simulink model "sun_point_unit_test"  (R2016b)
settings: Solver=VariableStepAuto  StartTime=0.0  StopTime=1000  MaxStep=0.01  RelTol=1e-4  EnableMultiTasking=on
undefined symbols (not defined in the file): fsw_params, sun_point_lib
libraries: aerolibutil x6, dspmathops x3, simulink x2
settings Model: Creator=Krish  LastModifiedBy=Taylor
settings DataIOCC: LimitDataPoints=on  SaveOutput=off  SaveTime=off
settings OptimizationCC: ExpressionDepthLimit=2147483647  LifeSpan=1
settings DebuggingCC: UnderspecifiedInitializationDetection=Classic  MergeDetectMultiDrivingBlocksExec=none  FcnCallInpInsideContextMsg=warning  AllowSymbolicDim=off  StateNameClashWarn=warning  SFUnexpectedBacktrackingDiag=warning  SFNoUnconditionalDefaultTransitionDiag=warning  SFExecutionAtInitializationDiag=none
settings GRTTargetCC: TargetLangStandard=C89/C90 (ANSI)  GeneratePreprocessorConditionals=Disable all  CombineOutputUpdateFcns=off  GRTInterface=on

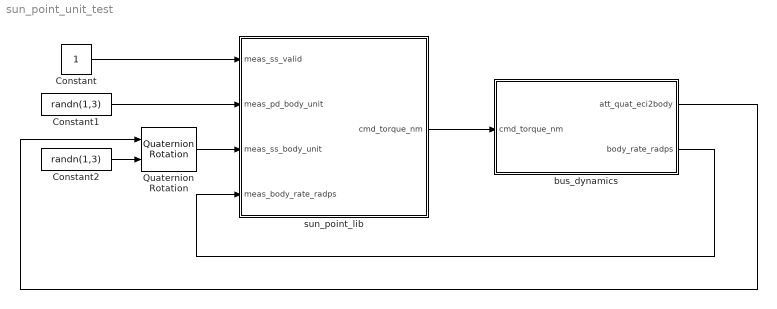
== system sun_point_unit_test ==
  Constant : Constant
  Constant1 : Constant  Value=randn(1,3)
  Constant2 : Constant  Value=randn(1,3)
  Quaternion Rotation : aerolibutil/Quaternion Rotation
  bus_dynamics : Subsystem
  sun_point_lib : Subsystem  AncestorBlock=sun_point_lib/sun_point_lib  TreatAsAtomicUnit=on
      settings: MinAlgLoopOccurrences=on  RTWFcnNameOpts=Use subsystem name  RTWFileNameOpts=Use subsystem name
  wires:
  sun_point_lib/1(cmd_torque_nm) -> bus_dynamics/1(cmd_torque_nm)
  Constant/1 -> sun_point_lib/1(meas_ss_valid)
  Constant1/1 -> sun_point_lib/2(meas_pd_body_unit)
  Quaternion Rotation/1 -> sun_point_lib/3(meas_ss_body_unit)
  Constant2/1 -> Quaternion Rotation/2
  bus_dynamics/1(att_quat_eci2body) -> Quaternion Rotation/1
  bus_dynamics/2(body_rate_radps) -> sun_point_lib/4(meas_body_rate_radps)

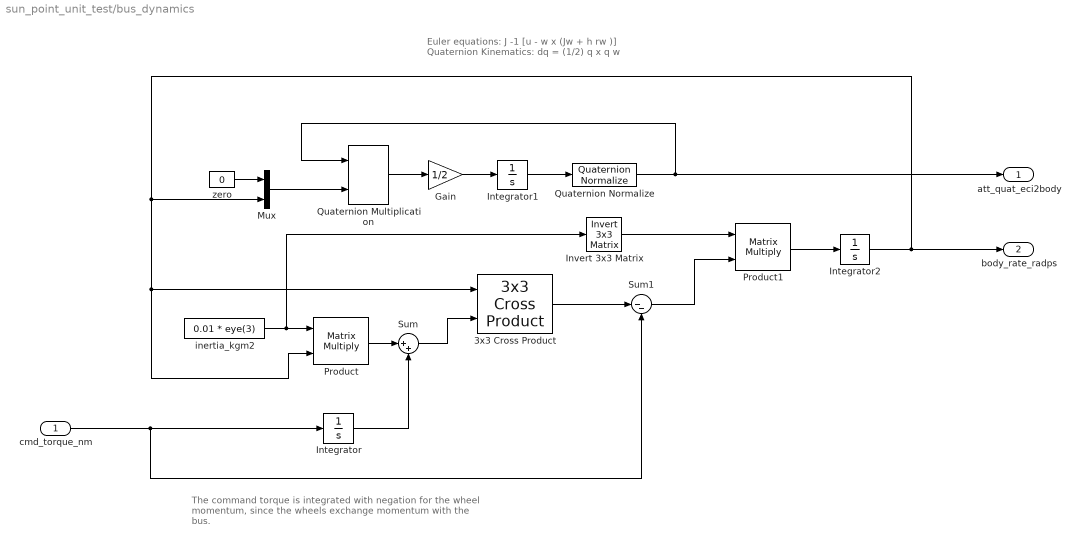
== system sun_point_unit_test/bus_dynamics ==
  note: Euler equations: J -1 [u - w x (Jw + h rw )]
      | Quaternion Kinematics: dq = (1/2) q x q w
  note: The command torque is integrated with negation for the wheel
      | momentum, since the wheels exchange momentum with the bus.
  cmd_torque_nm : Inport
  3x3 Cross Product : aerolibutil/3x3 Cross Product
  Gain : Gain  Gain=1/2
  Integrator : Integrator  InitialCondition=[0 0 0]
      settings: AttributesFormatString=IC: %<InitialCondition>
  Integrator1 : Integrator  InitialCondition=[1 0 0 0]
      settings: AttributesFormatString=IC: %<InitialCondition>
  Integrator2 : Integrator  InitialCondition=[0 0 0]
      settings: AttributesFormatString=IC: %<InitialCondition>
  Invert 3x3 Matrix : aerolibutil/Invert  3x3 Matrix
  Mux : Mux  Inputs=[1 3]
  Product : Product  Multiplication=Matrix(*)
  Product1 : Product  Multiplication=Matrix(*)
  Quaternion Multiplication : aerolibutil/Quaternion Multiplication
  Quaternion Normalize : aerolibutil/Quaternion Normalize
  Sum : Sum  Inputs=|++
  Sum1 : Sum  Inputs=|--
  inertia_kgm2 : Constant  Value=0.01 * eye(3)
  zero : Constant  Value=0
  att_quat_eci2body : Outport
  body_rate_radps : Outport  Port=2
  wires:
  Quaternion Normalize/1 -> att_quat_eci2body/1, Quaternion Multiplication/1
  Integrator2/1 -> body_rate_radps/1, 3x3 Cross Product/1, Product/2, Mux/2
  Product/1 -> Sum/1
  Sum/1 -> 3x3 Cross Product/2
  Integrator/1 -> Sum/2
  3x3 Cross Product/1 -> Sum1/1
  Integrator1/1 -> Quaternion Normalize/1
  zero/1 -> Mux/1
  Mux/1 -> Quaternion Multiplication/2
  Quaternion Multiplication/1 -> Gain/1
  Gain/1 -> Integrator1/1
  inertia_kgm2/1 -> Invert 3x3 Matrix/1, Product/1
  Invert 3x3 Matrix/1 -> Product1/1
  Sum1/1 -> Product1/2
  Product1/1 -> Integrator2/1
  cmd_torque_nm/1 -> Integrator/1, Sum1/2

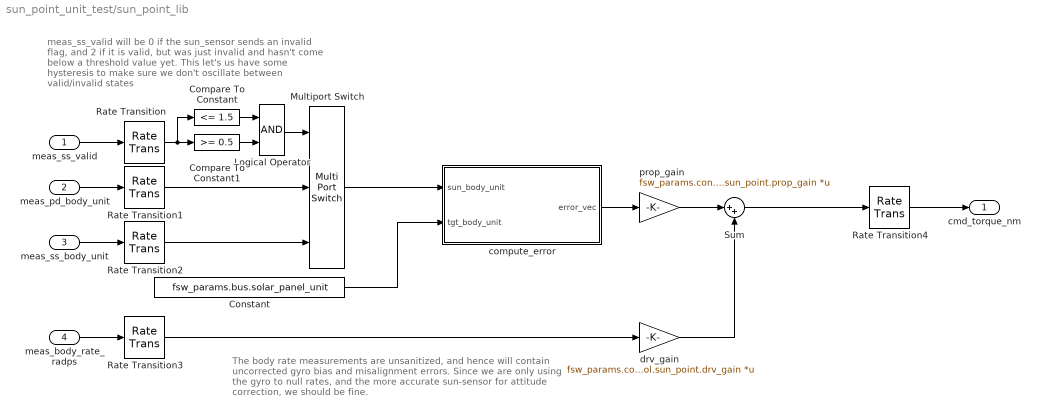
== system sun_point_unit_test/sun_point_lib ==
  note: The body rate measurements are unsanitized, and hence will contain
      | uncorrected gyro bias and misalignment errors. Since we are only using
      | the gyro to null rates, and the more accurate sun-sensor for attitude
      | correction, we should be fine.
  note: meas_ss_valid will be 0 if the sun_sensor sends an
      | invalid flag, and 2 if it is valid, but was just
      | invalid and hasn't come below a threshold value yet.
      | This let's us have some hysteresis to make sure we don't
      | oscillate between valid/invalid states
  meas_ss_valid : Inport
  meas_pd_body_unit : Inport  Port=2
  meas_ss_body_unit : Inport  Port=3
  meas_body_rate_radps : Inport  Port=4
  Compare To Constant : simulink/Logic and Bit Operations/Compare To Constant  relop=<=  const=1.5  OutDataTypeStr=boolean
  Compare To Constant1 : simulink/Logic and Bit Operations/Compare To Constant  relop=>=  const=0.5  OutDataTypeStr=boolean
  Constant : Constant  Value=fsw_params.bus.solar_panel_unit
  Logical Operator : Logic  AllPortsSameDT=off  OutDataTypeStr=boolean
  Multiport Switch : MultiPortSwitch  DataPortOrder=Zero-based contiguous  Inputs=2
  Rate Transition : RateTransition  X0=fsw_params.control.sun_point.ic.meas_ss_valid  OutPortSampleTime=fsw_params.control.sun_point.sample_time_s
  Rate Transition1 : RateTransition  X0=fsw_params.control.sun_point.ic.meas_pd_body_unit  OutPortSampleTime=fsw_params.control.sun_point.sample_time_s
  Rate Transition2 : RateTransition  X0=fsw_params.control.sun_point.ic.meas_ss_body_unit  OutPortSampleTime=fsw_params.control.sun_point.sample_time_s
  Rate Transition3 : RateTransition  X0=fsw_params.control.sun_point.ic.meas_body_rate_radps  OutPortSampleTime=fsw_params.control.sun_point.sample_time_s
  Rate Transition4 : RateTransition  X0=fsw_params.control.sun_point.ic.cmd_torque_nm  OutPortSampleTimeOpt=Inherit
  Sum : Sum  Inputs=|++
  compute_error : Subsystem
  drv_gain : Gain  Gain=fsw_params.control.sun_point.drv_gain  Multiplication=Matrix(K*u)
  prop_gain : Gain  Gain=fsw_params.control.sun_point.prop_gain  Multiplication=Matrix(K*u)
  cmd_torque_nm : Outport
  wires:
  Logical Operator/1 -> Multiport Switch/1
  Compare To Constant1/1 -> Logical Operator/2
  Compare To Constant/1 -> Logical Operator/1
  Rate Transition4/1 -> cmd_torque_nm/1
  Sum/1 -> Rate Transition4/1
  meas_body_rate_radps/1 -> Rate Transition3/1
  prop_gain/1 -> Sum/1
  meas_ss_body_unit/1 -> Rate Transition2/1
  Constant/1 -> compute_error/2(tgt_body_unit)
  drv_gain/1 -> Sum/2
  Rate Transition2/1 -> Multiport Switch/3
  meas_ss_valid/1 -> Rate Transition/1
  compute_error/1(error_vec) -> prop_gain/1
  meas_pd_body_unit/1 -> Rate Transition1/1
  Rate Transition3/1 -> drv_gain/1
  Rate Transition1/1 -> Multiport Switch/2
  Rate Transition/1 -> Compare To Constant1/1, Compare To Constant/1
  Multiport Switch/1 -> compute_error/1(sun_body_unit)

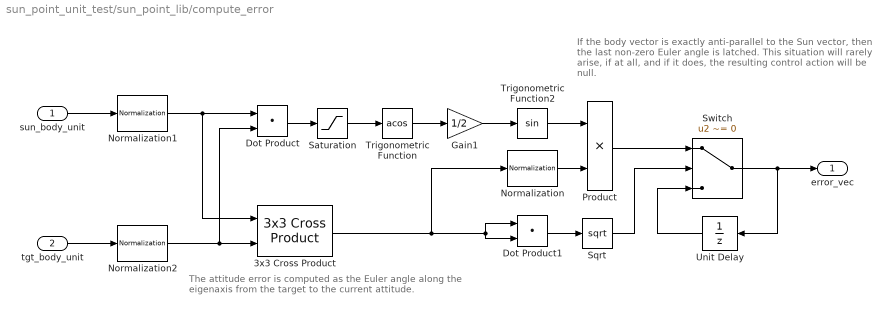
== system sun_point_unit_test/sun_point_lib/compute_error ==
  note: The attitude error is computed as the Euler angle along the
      | eigenaxis from the target to the current attitude.
  note: If the body vector is exactly anti-parallel to the Sun vector,
      | then the last non-zero Euler angle is latched. This situation
      | will rarely arise, if at all, and if it does, the resulting
      | control action will be null.
  sun_body_unit : Inport
  tgt_body_unit : Inport  Port=2
  3x3 Cross Product : aerolibutil/3x3 Cross Product
  Dot Product : DotProduct  InputSameDT=on  OutDataTypeStr=Inherit: Inherit via internal rule
  Dot Product1 : DotProduct  InputSameDT=on  OutDataTypeStr=Inherit: Inherit via internal rule
  Gain1 : Gain  Gain=1/2
  Normalization : dspmathops/Normalization  NormType=2-norm  Bias=1e-10  NormOver=Each column  Dimension=1  outputDataTypeStr=Inherit: Same as product output  outputLastDataTypeStr=Inherit: Same as product output  outputMin=[]  outputMax=[]  accumDataTypeStr=Inherit: Same as product output  accumLastDataTypeStr=Inherit: Same as product output  roundingMode=Floor  overflowMode=off
  Normalization1 : dspmathops/Normalization  NormType=2-norm  Bias=1e-10  NormOver=Each column  Dimension=1  outputDataTypeStr=Inherit: Same as product output  outputLastDataTypeStr=Inherit: Same as product output  outputMin=[]  outputMax=[]  accumDataTypeStr=Inherit: Same as product output  accumLastDataTypeStr=Inherit: Same as product output  roundingMode=Floor  overflowMode=off
  Normalization2 : dspmathops/Normalization  NormType=2-norm  Bias=1e-10  NormOver=Each column  Dimension=1  outputDataTypeStr=Inherit: Same as product output  outputLastDataTypeStr=Inherit: Same as product output  outputMin=[]  outputMax=[]  accumDataTypeStr=Inherit: Same as product output  accumLastDataTypeStr=Inherit: Same as product output  roundingMode=Floor  overflowMode=off
  Product : Product
  Saturation : Saturate  UpperLimit=1  LowerLimit=-1
      settings: AttributesFormatString=|
      | U: %<UpperLimit>
      | L: %<LowerLimit>
  Sqrt : Sqrt  SaturateOnIntegerOverflow=on
  Switch : Switch  Criteria=u2 ~= 0
  Trigonometric Function : Trigonometry  Operator=acos
  Trigonometric Function2 : Trigonometry
  Unit Delay : UnitDelay  InitialCondition=fsw_params.control.sun_point.ic.error_vec  SampleTime=-1
  error_vec : Outport
  wires:
  Normalization2/1 -> 3x3 Cross Product/2, Dot Product/2
  Normalization1/1 -> Dot Product/1, 3x3 Cross Product/1
  3x3 Cross Product/1 -> Normalization/1, Dot Product1/1, Dot Product1/2
  Dot Product1/1 -> Sqrt/1
  Sqrt/1 -> Switch/2
  Unit Delay/1 -> Switch/3
  Switch/1 -> Unit Delay/1, error_vec/1
  Dot Product/1 -> Saturation/1
  Trigonometric Function/1 -> Gain1/1
  Normalization/1 -> Product/2
  Gain1/1 -> Trigonometric Function2/1
  Saturation/1 -> Trigonometric Function/1
  sun_body_unit/1 -> Normalization1/1
  Product/1 -> Switch/1
  Trigonometric Function2/1 -> Product/1
  tgt_body_unit/1 -> Normalization2/1
